simulink model "X4_B"  (R2023b)
settings: Solver=VariableStepAuto  StartTime=0.0  StopTime=0.2  RelTol=1e-3
undefined symbols (not defined in the file or in its folder): Angle, Magnitude
libraries: spsCurrentMeasurementLib x2, spsRMSLib x2, spsSeriesRLCBranchLib x2, spsLinearTransformerLib x2, spsACVoltageSourceLib x1, spsVoltageMeasurementLib x1, sps_lib x1
settings Model: Creator=omdix  LastModifiedBy=omdix

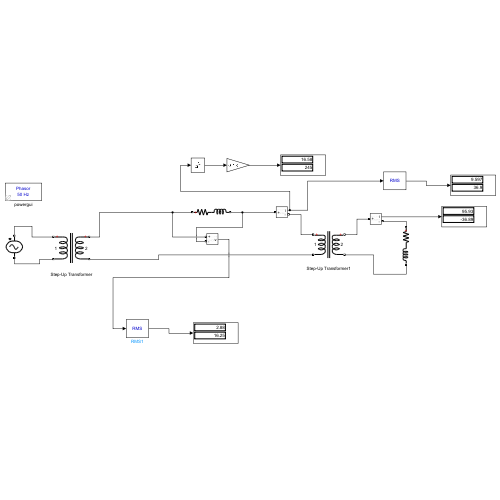
[thumbnail: Simulink's stored preview of the top-level diagram]
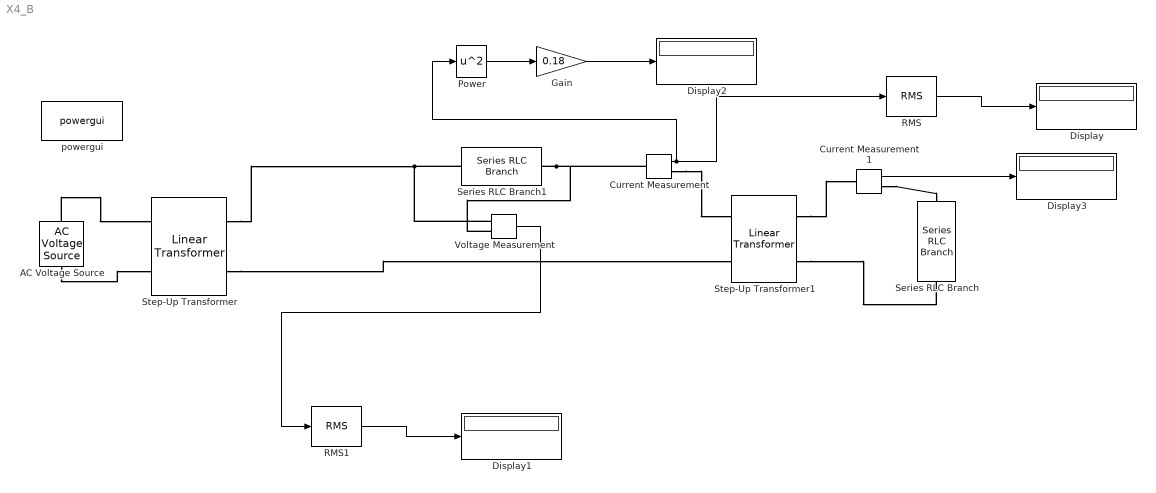
== system X4_B ==
  AC Voltage Source : spsACVoltageSourceLib/AC Voltage Source  Amplitude=480  Phase=0  Frequency=50  SampleTime=0  Measurements=None  BusType=swing  Pref=10e3  Qref=0  Qmin=-inf  Qmax=+inf
  Current Measurement : spsCurrentMeasurementLib/Current Measurement  PhasorSimulation=on  OutputType=Magnitude-Angle  PSBequivalent=0
  Current Measurement1 : spsCurrentMeasurementLib/Current Measurement  PhasorSimulation=on  OutputType=Magnitude-Angle  PSBequivalent=0
  Display{,1..3} (4 alike) : Display
  Gain : Gain  Gain=0.18
  Power : Math  Operator=square
  RMS : spsRMSLib/RMS  TrueRMS=on  Freq=50  RMSInit=120  Ts=0
  RMS1 : spsRMSLib/RMS  TrueRMS=on  Freq=50  RMSInit=120  Ts=0
  Series RLC Branch : spsSeriesRLCBranchLib/Series RLC Branch  LConnTagsString=__new0  RConnTagsString=__new0  BranchType=RL  Resistance=4  Inductance=3/314  SetiL0=off  InitialCurrent=0  Capacitance=1e-6  Setx0=off  InitialVoltage=0  Measurements=None
  Series RLC Branch1 : spsSeriesRLCBranchLib/Series RLC Branch  LConnTagsString=__new0  RConnTagsString=__new0  BranchType=RL  Resistance=0.18  Inductance=0.24/314  SetiL0=off  InitialCurrent=0  Capacitance=0  Setx0=off  InitialVoltage=0  Measurements=None
  Step-Up Transformer : spsLinearTransformerLib/Linear Transformer  UNITS=pu  NominalPower=[10000 50 ]  winding1=[480 0 0]  winding2=[4800 0 0]  ThreeWindings=off  winding3=[3.15e+05 0.0014142 0.056568]  RmLm=[707.08 707.12]  Measurements=None  DataType=off
  Step-Up Transformer1 : spsLinearTransformerLib/Linear Transformer  UNITS=pu  NominalPower=[10000 50 ]  winding1=[4800 0 0]  winding2=[480 0 0]  ThreeWindings=off  winding3=[3.15e+05 0.0014142 0.056568]  RmLm=[707.08 707.12]  Measurements=None  DataType=off
  Voltage Measurement : spsVoltageMeasurementLib/Voltage Measurement  PhasorSimulation=on  OutputType=Magnitude-Angle  PSBequivalent=0
  powergui : sps_lib/powergui  Priority=1  SimulationMode=Phasor  SampleTime=50e-6  frequency=50  Iterations=50  frequencyindice=50  Pbase=100e6  ErrMax=1e-4  UnitsV=kV  UnitsW=MW  buscounter=0  FunctionMessages=off  echomessages=off  EnableUseOfTLC=off  CurrentSourceSwitches=off  DisableSnubberDevices=off  DisableRonSwitches=off  DisableVfSwitches=off  DisplayEquations=off  AutomaticDiscreteSolvers=off  SolverType=Tustin/Backward Euler (TBE)  Interpol=off  ExternalGateDelay=off  methode=off  Ts=100  x0status=blocks  SPID=on  SwTol=0  HookPort=off  NonlinearTolerance=1e-4  nMaxIteration=100  ContinueOnMaxIteration=off  RestoreLinks=warning  ResistiveCurrentMeasurement=off  Frange=[0:2:500]  Ylog=off  Xlog=on  ShowGrid=off  save=off  variable=ZData  structure=0  ZoomFFT=off  StartTime=0.0  cycles=1  DisplayStyle=1  fundamental=60  FreqAxis=off  MaxFrequency=1000  frequencyindicesteady=1  RmsSteady=1  display=off
  wires:
  Power/1 -> Gain/1
  Current Measurement/1 -> Power/1, RMS/1
  RMS1/1 -> Display1/1
  Gain/1 -> Display2/1
  RMS/1 -> Display/1
  Voltage Measurement/1 -> RMS1/1
  Current Measurement1/1 -> Display3/1
  connections:
  Series RLC Branch1/RConn1 -- Current Measurement/LConn1 -- Voltage Measurement/LConn2
  Voltage Measurement/LConn1 -- Step-Up Transformer/RConn1 -- Series RLC Branch1/LConn1
  AC Voltage Source/RConn1 -- Step-Up Transformer/LConn1
  AC Voltage Source/LConn1 -- Step-Up Transformer/LConn2
  Current Measurement/RConn1 -- Step-Up Transformer1/LConn1
  Step-Up Transformer/RConn2 -- Step-Up Transformer1/LConn2
  Step-Up Transformer1/RConn1 -- Current Measurement1/LConn1
  Current Measurement1/RConn1 -- Series RLC Branch/LConn1
  Step-Up Transformer1/RConn2 -- Series RLC Branch/RConn1
